simulink model "Tuning_PID_0"  (R2019b)
settings: Solver=VariableStepAuto  StartTime=0.0  StopTime=10  RelTol=1e-3
settings Model: Creator=Rami  LastModifiedBy=Rami

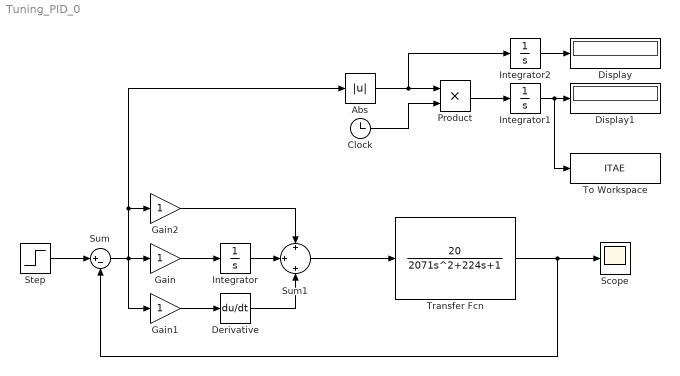
== system Tuning_PID_0 ==
  Abs : Abs
  Clock : Clock
  Derivative : Derivative
  Display : Display
  Display1 : Display
  Gain : Gain
  Gain1 : Gain
  Gain2 : Gain
  Integrator : Integrator
  Integrator1 : Integrator
  Integrator2 : Integrator
  Product : Product
  Scope : Scope
  Step : Step  SampleTime=0
  Sum : Sum  Inputs=|+-
  Sum1 : Sum  Inputs=+|+|+
  To Workspace : ToWorkspace  VariableName=ITAE  SampleTime=-1
  Transfer Fcn : TransferFcn  Numerator=[20]  Denominator=[2071 224 1]
  wires:
  Transfer Fcn/1 -> Scope/1, Sum/2
  Sum/1 -> Gain1/1, Gain/1, Abs/1, Gain2/1
  Gain2/1 -> Sum1/1
  Gain/1 -> Integrator/1
  Integrator/1 -> Sum1/2
  Gain1/1 -> Derivative/1
  Derivative/1 -> Sum1/3
  Sum1/1 -> Transfer Fcn/1
  Step/1 -> Sum/1
  Abs/1 -> Integrator2/1, Product/1
  Clock/1 -> Product/2
  Product/1 -> Integrator1/1
  Integrator2/1 -> Display/1
  Integrator1/1 -> To Workspace/1, Display1/1
